simulink model "P2"  (R2023b)
settings: Solver=VariableStepAuto  StartTime=0.0  StopTime=300  RelTol=1e-3
model workspace (MAT data in the model file):
  Q = 1000000000000
undefined symbols (not defined in the file): Continuous, Time
libraries: ctrlSharedLib x1
settings Model: Creator=ricar  LastModifiedBy=ricar

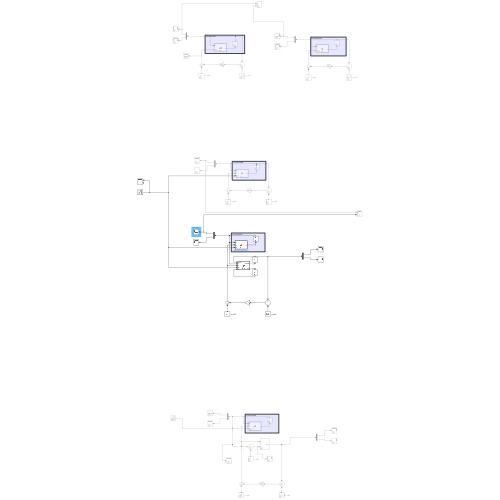
[thumbnail: Simulink's stored preview of the top-level diagram]
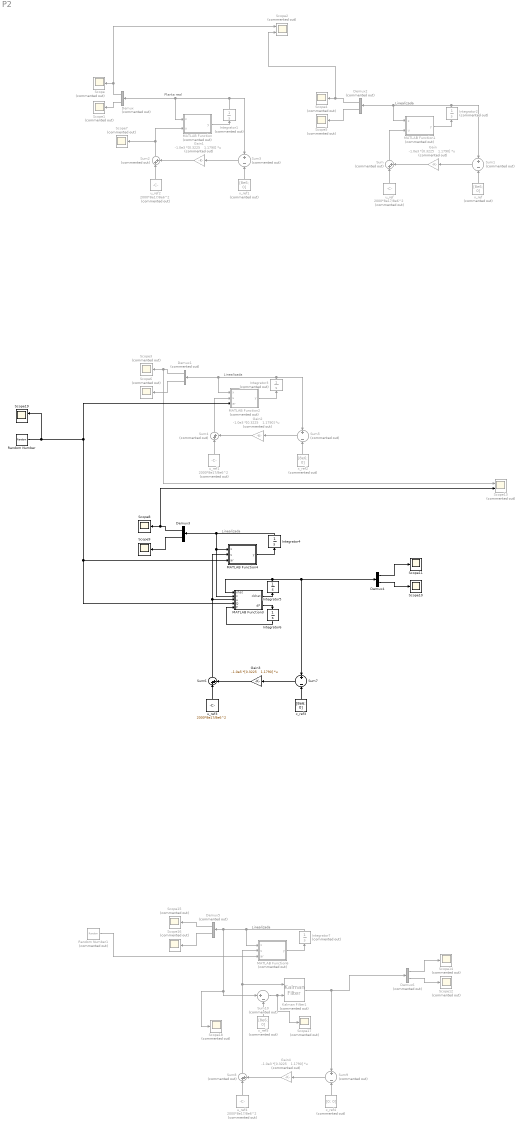
== system P2 ==
  note: Planta real
  note: Linealizada
  note: Linealizada
  note: Linealizada
  note: Linealizada
  Demux{,1..2,5..6} (5 alike) : Demux  Commented=on  Outputs=2
  Demux3 : Demux  Outputs=2
  Demux4 : Demux  Outputs=2
  Gain{,1..2,4} (4 alike) : Gain  Commented=on  Gain="-1.0e3 *[0.3225    1.1790]"  Multiplication=Matrix(K*u)
  Gain3 : Gain  Gain="-1.0e5 *[0.3225    1.1790]"  Multiplication=Matrix(K*u)
  Integrator1 : Integrator  Commented=on  InitialCondition=[8e6-1.5e6; -100]
  Integrator2 : Integrator  Commented=on  InitialCondition=[8e6-1.5e6; -100]
  Integrator3 : Integrator  Commented=on  InitialCondition=[8e6; 0]
  Integrator4 : Integrator  InitialCondition=[8e6; 0]
  Integrator5 : Integrator  InitialCondition=[8e6; 0]
  Integrator6 : Integrator  InitialCondition=eye(2)
  Integrator7 : Integrator  Commented=on  InitialCondition=[8e6; 0]
  Kalman Filter1 : ctrlSharedLib/Kalman Filter  Commented=on  TimeDomain=Continuous-Time  UseCurrentEstimator=on  ModelSource=Individual A, B, C, D matrices  ModelSourceVariable=ss(0.95,1,1,0,1)  A=[0 1; 2*8e17/8e6^3 0]  B=[0;1/2000]  C=eye(2)  D=0  NumberOfStates=1  NumberOfInputs=1  NumberOfOutputs=1  InitialEstimateSource=Dialog  X0=[0;0]  P0=10  UseK=off  UseGH=on  NumberOfProcessNoiseInputs=1  G=[0 0;0 1]  TimeInvariantG=on  H=0  TimeInvariantH=on  Q=[0 0;0 1e12]  TimeInvariantQ=on  R=[1e-6 0;0 1e-6]  TimeInvariantR=on  N=0  TimeInvariantN=on  AddInputPort=on  AddEnablePort=off  OutputEstimatedY=off  OutputP=off  Ts=-1
  MATLAB Function : MATLAB Function  Commented=on  TreatAsAtomicUnit=on
  MATLAB Function1 : MATLAB Function  Commented=on  TreatAsAtomicUnit=on
  MATLAB Function2 : MATLAB Function  Commented=on  TreatAsAtomicUnit=on
  MATLAB Function3 : MATLAB Function  TreatAsAtomicUnit=on
  MATLAB Function4 : MATLAB Function  TreatAsAtomicUnit=on
  MATLAB Function6 : MATLAB Function  Commented=on  TreatAsAtomicUnit=on
  Random Number : RandomNumber  Variance=6.5e14  SampleTime=1e-4
  Random Number1 : RandomNumber  Commented=on  Variance=1e12  SampleTime=0.1
  Scope{,1,3..7,12,14..18} (13 alike) : Scope  Commented=on
  Scope{8..11} (4 alike) : Scope
  Scope13 : Scope  Commented=on  NumInputPorts=2
  Scope19 : Scope  NumInputPorts=2
  Scope2 : Scope  Commented=on  NumInputPorts=2
  Sum{,2,4,8} (4 alike) : Sum  Commented=on  Inputs=|++
  Sum{1,3,5,9} (4 alike) : Sum  Commented=on  Inputs=+|-
  Sum10 : Sum  Commented=on  Inputs=|+-
  Sum6 : Sum  Inputs=|++
  Sum7 : Sum  Inputs=+|-
  u_ref{,1..2,4} (4 alike) : Constant  Commented=on  Value=2000*8e17/8e6^2
  u_ref3 : Constant  Value=2000*8e17/8e6^2
  x_ref{,1..2,5} (4 alike) : Constant  Commented=on  Value=[8e6; 0]
  x_ref3 : Constant  Value=[8e6; 0]
  x_ref4 : Constant  Commented=on  Value=[0; 0]
  wires:
  Demux/1 -> Scope2/1, Scope/1
  Demux/2 -> Scope1/1
  MATLAB Function/1(y) -> Integrator1/1
  Integrator1/1 -> Sum3/1, MATLAB Function/1(x), Demux/1
  Demux2/2 -> Scope5/1
  Gain/1 -> Sum/2
  Demux2/1 -> Scope2/2, Scope4/1
  MATLAB Function1/1(y) -> Integrator2/1
  Sum/1 -> MATLAB Function1/2(u)
  Sum1/1 -> Gain/1
  x_ref/1 -> Sum1/2
  u_ref/1 -> Sum/1
  Integrator2/1 -> Sum1/1, MATLAB Function1/1(x), Demux2/1
  u_ref2/1 -> Sum2/1
  x_ref1/1 -> Sum3/2
  Sum3/1 -> Gain1/1
  Gain1/1 -> Sum2/2
  Sum2/1 -> Scope7/1, MATLAB Function/2(u)
  Integrator3/1 -> Sum5/1, MATLAB Function2/1(x), Demux1/1
  u_ref1/1 -> Sum4/1
  x_ref2/1 -> Sum5/2
  MATLAB Function2/1(y) -> Integrator3/1
  Sum4/1 -> MATLAB Function2/2(u)
  Demux1/2 -> Scope6/1
  Demux1/1 -> Scope13/1, Scope3/1
  Gain2/1 -> Sum4/2
  Sum5/1 -> Gain2/1
  MATLAB Function4/1(y) -> Integrator4/1
  Sum7/1 -> Gain3/1
  Random Number/1 -> Scope19/1, MATLAB Function2/3(ar), MATLAB Function3/4(Q), MATLAB Function4/3(ar)
  Gain3/1 -> Sum6/2
  Sum6/1 -> MATLAB Function3/3(u), MATLAB Function4/2(u)
  Demux3/1 -> Scope13/2, Scope8/1
  Demux3/2 -> Scope9/1
  Integrator4/1 -> MATLAB Function3/2(x), MATLAB Function4/1(x), Demux3/1
  u_ref3/1 -> Sum6/1
  x_ref3/1 -> Sum7/2
  MATLAB Function3/1(dxhat) -> Integrator5/1
  Integrator5/1 -> Sum7/1, Demux4/1, MATLAB Function3/1(xhat)
  Demux4/1 -> Scope11/1
  Demux4/2 -> Scope10/1
  MATLAB Function3/2(dP) -> Integrator6/1
  Integrator6/1 -> MATLAB Function3/5(P)
  Random Number1/1 -> MATLAB Function6/3(ar)
  Demux6/2 -> Scope12/1
  Demux6/1 -> Scope14/1
  x_ref4/1 -> Sum9/2
  Integrator7/1 -> MATLAB Function6/1(x), Scope18/1, Sum10/1, Demux5/1
  u_ref4/1 -> Sum8/1
  Demux5/2 -> Scope16/1
  Sum8/1 -> Kalman Filter1/1, MATLAB Function6/2(u)
  Sum9/1 -> Gain4/1
  Gain4/1 -> Sum8/2
  Demux5/1 -> Scope15/1
  MATLAB Function6/1(y) -> Integrator7/1
  Kalman Filter1/1 -> Sum9/1, Demux6/1
  x_ref5/1 -> Sum10/2
  Sum10/1 -> Scope17/1, Kalman Filter1/2

== matlab function P2/MATLAB Function1 ==
  data: x input; u input; y output
function y = fcn(x,u)
A = [0 1; 2*8e17/8e6^3 0];
B = [0;1/2000];
%C = eye(2);

x_ref = [8e6; 0];
u_ref = 2000*8e17/8e6^2;

if x(1) <= 6378e3
    dx = [0;0];
else
dx = A*(x-x_ref) + B*(u-u_ref);
end


y = dx;

== matlab function P2/MATLAB Function ==
  data: x input; u input; y output
function y = fcn(x,u)

if x(1) <= 6378e3
    dx = [0;0];
else
dx = [x(2);-8e17/(x(1))^2+u/2000];
end


y = dx;

== matlab function P2/MATLAB Function2 ==
  data: x input; u input; y output; ar input
function y = fcn(x,u,ar)
A = [0 1; 2*8e17/8e6^3 0];
B = [0;1/2000];
%C = eye(2);

x_ref = [8e6; 0];
u_ref = 2000*8e17/8e6^2;

if x(1) <= 6378e3
    dx = [0;0];
else
dx = A*(x-x_ref) + B*(u-u_ref)+[0;1]*ar;
end


y = dx;

== matlab function P2/MATLAB Function3 ==
  data: xhat input; x input; u input; Q input; dxhat output; P input; dP output
function [dxhat,dP] = fcn(xhat,x,u,Q,P)

A = [0 1; 2*8e17/8e6^3 0];
B = [0;1/2000];
C = eye(2);

L = [0    0
    0    316230];

x_ref = [8e6; 0];
u_ref = 2000*8e17/8e6^2;

Q_k = [0, Q];                  % Ruido de proceso
R_k = 1e-6*[1 1];                  % Ruido de medicion

%Filtro de Kalman
dxhat_t = A*(xhat-x_ref) + B*(u-u_ref) + L*(C*x - C*xhat);
P = A*P*A'+Q_k;
e = xhat - x;
K = P*C'*inv(C*P*C'+R_k);
dxhat = dxhat_t - K*e;
dP = K*C*P;

== matlab function P2/MATLAB Function4 ==
  data: x input; u input; y output; ar input
function y = fcn(x,u,ar)
A = [0 1; 2*8e17/8e6^3 0];
B = [0;1/2000];
%C = eye(2);

x_ref = [8e6; 0];
u_ref = 2000*8e17/8e6^2;

if x(1) <= 6378e3
    dx = [0;0];
else
dx = A*(x-x_ref) + B*(u-u_ref)+[0;1]*ar;
end


y = dx;

== matlab function P2/MATLAB Function6 ==
  data: x input; u input; y output; ar input
function y = fcn(x,u,ar)
A = [0 1; 2*8e17/8e6^3 0];
B = [0;1/2000];
%C = eye(2);

x_ref = [8e6; 0];
u_ref = 2000*8e17/8e6^2;

if x(1) <= 6378e3
    dx = [0;0];
else
dx = A*(x-x_ref) + B*(u-u_ref)+[0;1]*ar;
end


y = dx;
